simulink model "test2"  (R2015a)
settings: Solver=ode3  SolverMode=SingleTasking  StartTime=0.0  StopTime=inf  RelTol=1e-3
settings Model: ExtModeTrigDuration=2  Creator=kkhoo  LastModifiedBy=kkhoo
settings OptimizationCC: OptimizeModelRefInitCode=on  LifeSpan=1
settings DebuggingCC: UnderspecifiedInitializationDetection=Classic  MergeDetectMultiDrivingBlocksExec=none
settings HardwareCC: ProdBitPerInt=16  ProdBitPerPointer=8  ProdIntDivRoundTo=Zero  ProdEndianess=LittleEndian  ProdWordSize=8  ProdHWDeviceType=Atmel->AVR
settings RTWCC: SystemTargetFile=realtime.tlc  GenerateMakefile=off  TemplateMakefile=realtime.tmf  Description=Run on Target Hardware  RTWVerbose=off  CustomSource=src/Engduino.h src/engduino_wrappers.cpp
settings ERTTargetCC: CombineOutputUpdateFcns=off  ExtModeTransport=3  ExtModeMexFile=ext_serial_win32_comm_rtt  ExtModeMexArgs=0 1 9600  ERTSrcFileBannerTemplate=realtime_code_template.cgt  ERTHdrFileBannerTemplate=realtime_code_template.cgt  ERTDataSrcFileTemplate=realtime_code_template.cgt  ERTDataHdrFileTemplate=realtime_code_template.cgt  ERTCustomFileTemplate=realtime_file_process.tlc

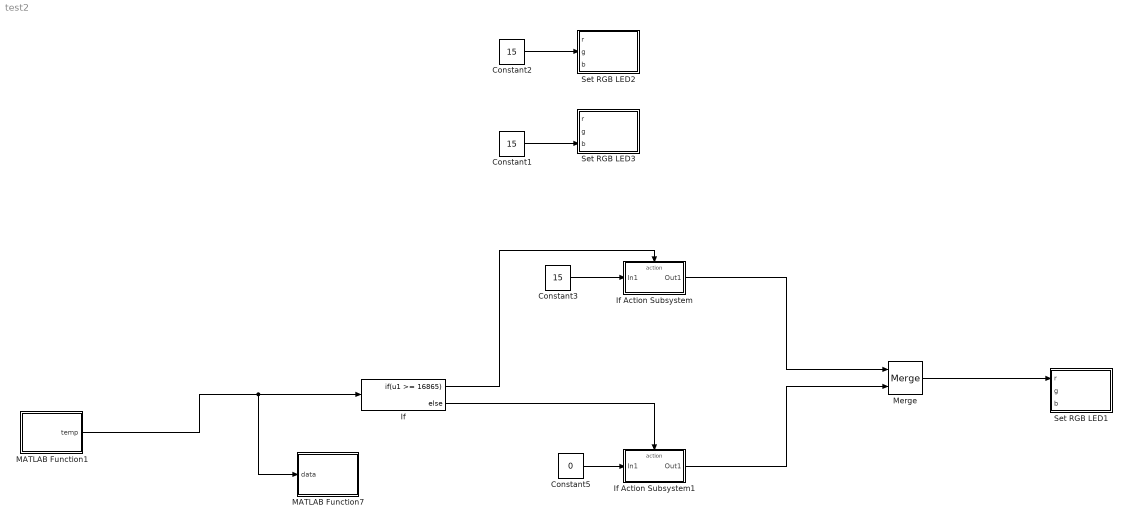
== system test2 ==
  Constant1 : Constant  Value=15  OutDataTypeStr=Inherit: Inherit via back propagation
  Constant2 : Constant  Value=15  OutDataTypeStr=Inherit: Inherit via back propagation
  Constant3 : Constant  Value=15  OutDataTypeStr=uint8
  Constant5 : Constant  Value=0  OutDataTypeStr=uint8
  If : If  IfExpression=u1 >= 16865
  If Action Subsystem : Subsystem  TreatAsAtomicUnit=on
  If Action Subsystem1 : Subsystem  TreatAsAtomicUnit=on
  MATLAB Function1 : MATLAB Function  LoadFcn=|  TreatAsAtomicUnit=on  mask(Thermistor){}
      | set_param(gcs, 'CustomSource', strjoin(unique([strsplit(get_param(gcs, 'CustomSource')) ...
      |  'src/engduino_wrappers.cpp' 'src/Engduino.h'])));
      mask help: Outputs the temperature in milli degrees celsius.
  MATLAB Function7 : MATLAB Function  LoadFcn=|  TreatAsAtomicUnit=on  mask(Serial Transmission){}
      | set_param(gcs, 'CustomSource', strjoin(unique([strsplit(get_param(gcs, 'CustomSource')) ...
      |  'src/engduino_wrappers.cpp' 'src/Engduino.h'])));
      mask help: Output data as uint8_t through serial
  Merge : Merge
  Set RGB LED1 : MATLAB Function  LoadFcn=|  TreatAsAtomicUnit=on  mask(RGB LED){led_index=0}
      | set_param(gcs, 'CustomSource', strjoin(unique([strsplit(get_param(gcs, 'CustomSource')) ...
      |  'src/engduino_wrappers.cpp' 'src/Engduino.h'])));
      mask prompts: led_index "LED index"
      mask help:
      | Control the Red, Green and Blue color values of the LED specified by the LED index parameter.
      | Both the LED index and the three color values are of type uint8 and must be in the range 0-15.
      settings: AttributesFormatString=LED %<led_index>
  Set RGB LED2 : MATLAB Function  LoadFcn=|  TreatAsAtomicUnit=on  mask(RGB LED){led_index=1}
      | set_param(gcs, 'CustomSource', strjoin(unique([strsplit(get_param(gcs, 'CustomSource')) ...
      |  'src/engduino_wrappers.cpp' 'src/Engduino.h'])));
      mask prompts: led_index "LED index"
      mask help:
      | Control the Red, Green and Blue color values of the LED specified by the LED index parameter.
      | Both the LED index and the three color values are of type uint8 and must be in the range 0-15.
      settings: AttributesFormatString=LED %<led_index>
  Set RGB LED3 : MATLAB Function  LoadFcn=|  TreatAsAtomicUnit=on  mask(RGB LED){led_index=2}
      | set_param(gcs, 'CustomSource', strjoin(unique([strsplit(get_param(gcs, 'CustomSource')) ...
      |  'src/engduino_wrappers.cpp' 'src/Engduino.h'])));
      mask prompts: led_index "LED index"
      mask help:
      | Control the Red, Green and Blue color values of the LED specified by the LED index parameter.
      | Both the LED index and the three color values are of type uint8 and must be in the range 0-15.
      settings: AttributesFormatString=LED %<led_index>
  wires:
  Constant2/1 -> Set RGB LED2/2(g)
  Constant1/1 -> Set RGB LED3/3(b)
  If/1 -> If Action Subsystem/Action
  If/2 -> If Action Subsystem1/Action
  MATLAB Function1/1(temp) -> MATLAB Function7/1(data), If/1
  Constant5/1 -> If Action Subsystem1/1(In1)
  Merge/1 -> Set RGB LED1/1(r)
  Constant3/1 -> If Action Subsystem/1(In1)
  If Action Subsystem/1(Out1) -> Merge/1
  If Action Subsystem1/1(Out1) -> Merge/2

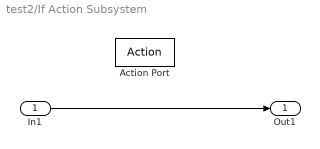
== system test2/If Action Subsystem ==
  In1 : Inport
  Action Port : ActionPort  ActionType=then
  Out1 : Outport  OutDataTypeStr=uint8
  wires:
  In1/1 -> Out1/1

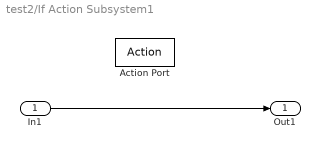
== system test2/If Action Subsystem1 ==
  In1 : Inport
  Action Port : ActionPort  ActionType=else
  Out1 : Outport  OutDataTypeStr=uint8
  wires:
  In1/1 -> Out1/1

== matlab function test2/Set RGB LED3 ==
  data: led_index parameter uint8 [0..15]; r input uint8 [0..15]; g input uint8 [0..15]; b input uint8 [0..15]
function rgb_led(led_index, r, g, b)

if strcmp(coder.target, 'rtw')
    coder.ceval('rgb_leds_wrapper', led_index, r, g, b);
end

== matlab function test2/Set RGB LED1 ==
  data: led_index parameter uint8 [0..15]; r input uint8 [0..15]; g input uint8 [0..15]; b input uint8 [0..15]
function rgb_led(led_index, r, g, b)

if strcmp(coder.target, 'rtw')
    coder.ceval('rgb_leds_wrapper', led_index, r, g, b);
end

== matlab function test2/Set RGB LED2 ==
  data: led_index parameter uint8 [0..15]; r input uint8 [0..15]; g input uint8 [0..15]; b input uint8 [0..15]
function rgb_led(led_index, r, g, b)

if strcmp(coder.target, 'rtw')
    coder.ceval('rgb_leds_wrapper', led_index, r, g, b);
end

== matlab function test2/MATLAB Function7 ==
  data: data input
function print_data(data)

if strcmp(coder.target, 'rtw')
    coder.ceval('print_data_serial_wrapper', data);
end

== matlab function test2/MATLAB Function1 ==
  data: temp output
function temp = thermistor()

temp = 0.0;

if strcmp(coder.target, 'rtw')
    temp = coder.ceval('thermistor_wrapper');
end
